simulink model "counter"  (R2020b)
settings: Solver=VariableStepAuto  StartTime=0.0  StopTime=60.0  RelTol=1e-3
settings Model: Creator=Admin  LastModifiedBy=Admin

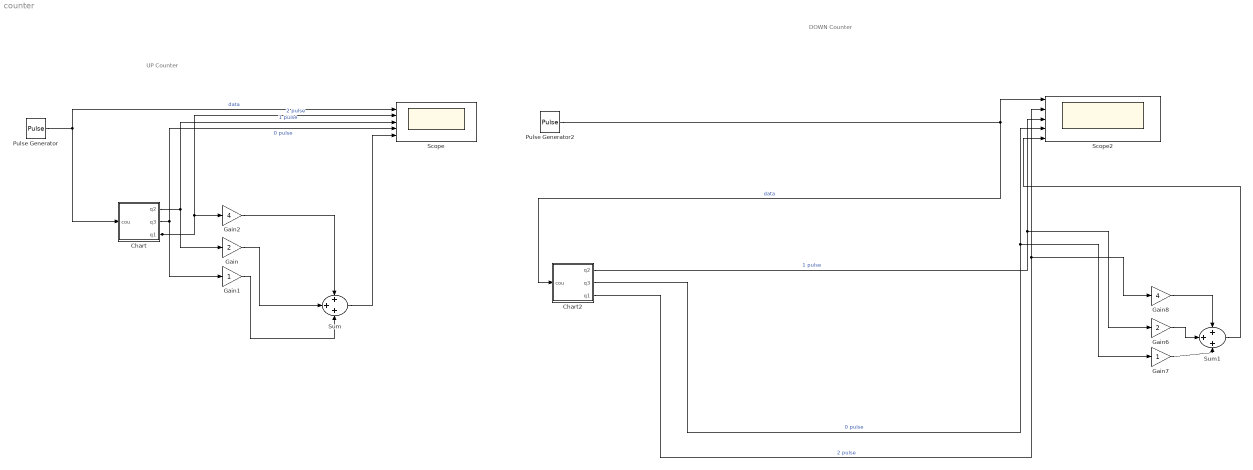
== system counter ==
  note: UP Counter
  note: DOWN Counter
  Chart : Stateflow chart  TreatAsAtomicUnit=on
  Chart2 : Stateflow chart  TreatAsAtomicUnit=on
  Gain : Gain  Gain=2
  Gain1 : Gain
  Gain2 : Gain  Gain=4
  Gain6 : Gain  Gain=2
  Gain7 : Gain
  Gain8 : Gain  Gain=4
  Pulse Generator : DiscretePulseGenerator  PulseType=Time based  Period=10  PulseWidth=50
  Pulse Generator2 : DiscretePulseGenerator  PulseType=Time based  Period=10  PulseWidth=50
  Scope : Scope  NumInputPorts=5
  Scope2 : Scope  NumInputPorts=5
  Sum : Sum  Inputs=+++
  Sum1 : Sum  Inputs=+++
  wires:
  Gain1/1 -> Sum/3
  Chart/1(q2) -> Gain/1, Scope/3  "1 pulse"
  Gain2/1 -> Sum/1
  Chart/3(q1) -> Scope/2, Gain2/1  "2 pulse"
  Gain/1 -> Sum/2
  Sum/1 -> Scope/5
  Chart/2(q3) -> Scope/4, Gain1/1  "0 pulse"
  Pulse Generator/1 -> Chart/1(cou), Scope/1  "data"
  Gain7/1 -> Sum1/3
  Chart2/1(q2) -> Gain6/1, Scope2/3  "1 pulse"
  Gain8/1 -> Sum1/1
  Gain6/1 -> Sum1/2
  Chart2/2(q3) -> Gain7/1, Scope2/4  "0 pulse"
  Sum1/1 -> Scope2/5
  Chart2/3(q1) -> Gain8/1, Scope2/2  "2 pulse"
  Pulse Generator2/1 -> Chart2/1(cou), Scope2/1  "data"

== stateflow chart counter/Chart2 ==
  state a_case1
    entry:
    q1=0;
    q2=0;
    q3=0;
  state a_case5
    entry:
    q1=1;
    q2=0;
    q3=0;
  state entry_
    q1=0;
    q2=0;
    q3=0;
  state entry_1
    q1=0;
    q2=0;
    q3=1;
  state a_case2
    entry:
    q1=0;
    q2=0;
    q3=1;
  state entry_4
    q1=1;
    q2=0;
    q3=0;
  state entry_2
    q1=0;
    q2=1;
    q3=0;
  state a_case4
    entry:
    q1=0;
    q2=1;
    q3=1;
  state a_case3
    entry:
    q1=0;
    q2=1;
    q3=0;
  state entry_3
    q1=0;
    q2=1;
    q3=1;
  (default) -> state47
  a_case1 -> state47 : [cou==0]
  state47 -> a_case5 : [cou==1]
  state43 -> a_case1 : [cou==1]
  a_case5 -> state41 : [cou==0]
  a_case2 -> state43 : [cou==0]
  state44 -> a_case2 : [cou==1]
  state41 -> a_case4 : [cou==1]
  a_case3 -> state44 : [cou==0]
  a_case4 -> state46 : [cou==0]
  state46 -> a_case3 : [cou==1]
  data: q2 output; q3 output; q1 output; cou input

== stateflow chart counter/Chart ==
  state a_case1
    entry:
    q1=0;
    q2=0;
    q3=0;
  state entry_
    q1=0;
    q2=0;
    q3=0;
  state a_case5
    entry:
    q1=1;
    q2=0;
    q3=0;
  state entry_1
    q1=0;
    q2=0;
    q3=1;
  state a_case2
    entry:
    q1=0;
    q2=0;
    q3=1;
  state entry_4
    q1=1;
    q2=0;
    q3=0;
  state entry_2
    q1=0;
    q2=1;
    q3=0;
  state a_case4
    entry:
    q1=0;
    q2=1;
    q3=1;
  state entry_3
    q1=0;
    q2=1;
    q3=1;
  state a_case3
    entry:
    q1=0;
    q2=1;
    q3=0;
  (default) -> state47
  state47 -> a_case1 : [cou==0]
  a_case5 -> state47 : [cou==1]
  a_case1 -> state43 : [cou==1]
  state41 -> a_case5 : [cou==0]
  state43 -> a_case2 : [cou==0]
  a_case2 -> state44 : [cou==1]
  a_case4 -> state41 : [cou==1]
  state44 -> a_case3 : [cou==0]
  state46 -> a_case4 : [cou==0]
  a_case3 -> state46 : [cou==1]
  data: q2 output; q3 output; q1 output; cou input
